simulink model "Sum8"  (R2020b)
settings: Solver=VariableStepAuto  StartTime=0.0  StopTime=10.0  RelTol=1e-3
settings Model: Creator=Aradhana desai  LastModifiedBy=Aradhana desai

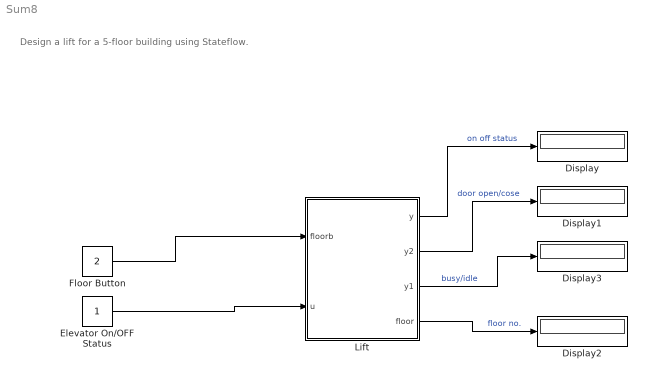
== system Sum8 ==
  note: Design a lift for a 5-floor building using Stateflow.
  Display{,1..3} (4 alike) : Display
  Elevator On/OFF Status : Constant
  Floor Button : Constant  Value=2
  Lift : Stateflow chart  TreatAsAtomicUnit=on
  wires:
  Floor Button/1 -> Lift/1(floorb)
  Elevator On/OFF Status/1 -> Lift/2(u)
  Lift/1(y) -> Display/1  "on off status"
  Lift/2(y2) -> Display1/1  "door open/cose"
  Lift/3(y1) -> Display3/1  "busy/idle"
  Lift/4(floor) -> Display2/1  "floor no."

== stateflow chart Sum8/Lift ==
  state Elevator_on
    entry: y=1;
    note: [floorb<floor]{y1= 1 }
    state DOWN
      entry:
      floor=floor-1;
    state Delay1
      entry:
      floor=floor-1;
    state Idle_state
      entry: y1=0;
    state UP
      entry:
      floor=floor+1;
    state Delay
      entry:
      floor=floor+1;
    state Door_open1
      entry:
      y2=1;
    state Door_close1
      entry:
      y2=0;
    state Door_open
      entry:
      y2=1;
    state Door_close
      entry:
      y2=0;
    (default) -> Idle_state
    DOWN -> Delay1 [order 1] : [floorb<floor]
    Idle_state -> DOWN [order 2]
    Delay1 -> DOWN [order 1] : [floorb<floor]
    Idle_state -> UP [order 1] : [floorb>floor]{y1=1}
    DOWN -> Door_open1 [order 2] : [floorb==floor]
    Delay1 -> Door_open1 [order 2] : [floor==floorb]
    Delay -> UP [order 1] : [floorb>floor]
    UP -> Delay [order 1] : [floorb>floor]
    Door_open1 -> Door_close1 : [after(5,sec)]
    UP -> Door_open [order 2] : [floorb==floor]
    Delay -> Door_open [order 2] : [floor==floorb]
    Door_open -> Door_close : [after(5,sec)]
  state Elevator_off
    entry: y=0;
  (default) -> Elevator_on
  Elevator_on -> Elevator_off : [u==0]
  Elevator_off -> Elevator_on : [u==1]
  data: floorb input; u input; y output; y2 output; y1 output; floor output
